simulink model "model_1"  (R2023b)
settings: Solver=VariableStepAuto  StartTime=0.0  StopTime=10.0  RelTol=1e-3
settings Model: Creator=Lenovo  LastModifiedBy=Lenovo
settings DataIOCC: ReturnWorkspaceOutputs=off

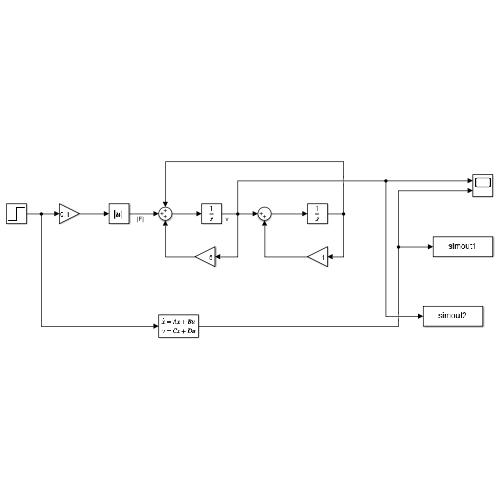
[thumbnail: Simulink's stored preview of the top-level diagram]
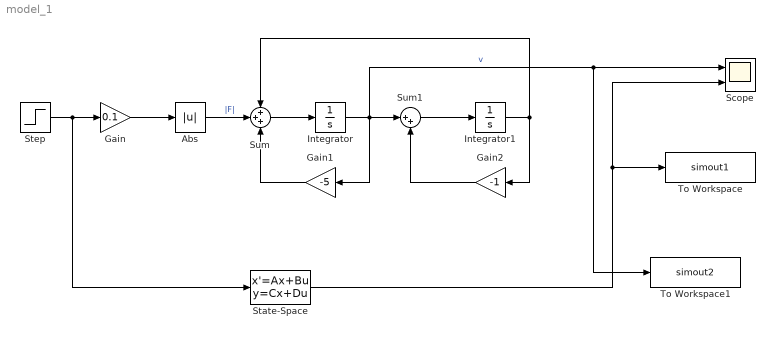
== system model_1 ==
  Abs : Abs  SaturateOnIntegerOverflow=off
  Gain : Gain  Gain=0.1
  Gain1 : Gain  Gain=-5
  Gain2 : Gain  Gain=-1
  Integrator : Integrator
  Integrator1 : Integrator
  Scope : Scope  NumInputPorts=2
  State-Space : StateSpace  A=[-5, 1;1, -1]  B=[0.1;0]  C=[1, 0]  D=0  InitialCondition=0
  Step : Step  SampleTime=0
  Sum : Sum  Inputs=+++
  Sum1 : Sum  Inputs=|++
  To Workspace : ToWorkspace  VariableName=simout1  SaveFormat=Timeseries  SampleTime=-1
  To Workspace1 : ToWorkspace  VariableName=simout2  SaveFormat=Timeseries  SampleTime=-1
  wires:
  Step/1 -> State-Space/1, Gain/1
  Gain/1 -> Abs/1
  Abs/1 -> Sum/2  "|F|"
  Sum/1 -> Integrator/1
  Sum1/1 -> Integrator1/1
  Integrator1/1 -> Gain2/1, Sum/1
  Integrator/1 -> To Workspace1/1, Scope/1, Gain1/1, Sum1/1  "v"
  Gain1/1 -> Sum/3
  Gain2/1 -> Sum1/2
  State-Space/1 -> To Workspace/1, Scope/2
